simulink model "prob3"  (R2020b)
settings: Solver=VariableStepAuto  StartTime=0.0  StopTime=10.0  RelTol=1e-3
settings Model: Creator=nadee  LastModifiedBy=nadee

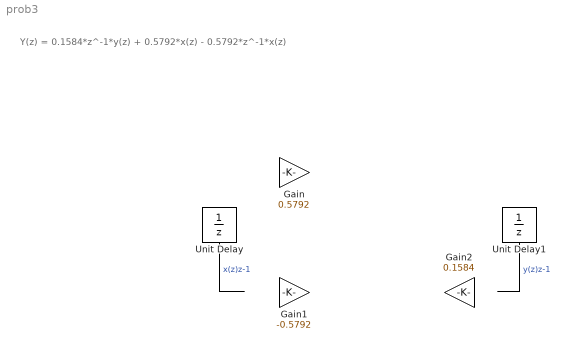
== system prob3 ==
  note: Y(z) = 0.1584*z^-1*y(z) + 0.5792*x(z) - 0.5792*z^-1*x(z)
  Gain : Gain  Gain=0.5792
  Gain1 : Gain  Gain=-0.5792
  Gain2 : Gain  Gain=0.1584
  Unit Delay : UnitDelay  SampleTime=-1  HasFrameUpgradeWarning=on
  Unit Delay1 : UnitDelay  SampleTime=-1  HasFrameUpgradeWarning=on
  wires:
  Unit Delay/1 -> ?  "x(z)z-1"
  ? -> Gain/1  "x(z)"
  ? -> Unit Delay1/1  "y(z)"
  Unit Delay1/1 -> ?  "y(z)z-1"
